simulink model "Damaper"  (R2024b)
settings: Solver=VariableStepAuto  StartTime=0.0  StopTime=10.0  RelTol=1e-3
values from neighbouring files (symbols this model uses):
  b = 10    [Damper.m]
  k = 400    [Damper.m]
  m = massValues(i)    [Damper.m]
  x0 = 1    [Damper.m]
settings Model: Creator=Ahmad  LastModifiedBy=Ahmad

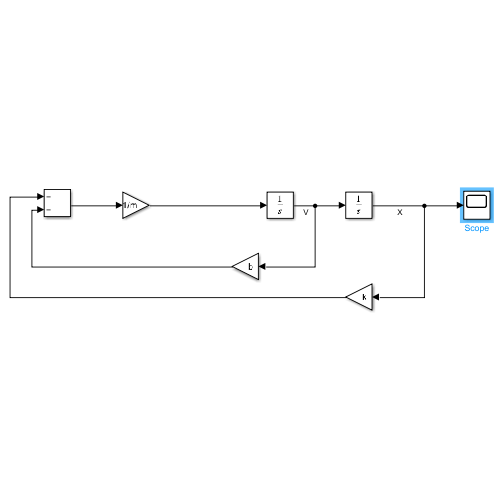
[thumbnail: Simulink's stored preview of the top-level diagram]
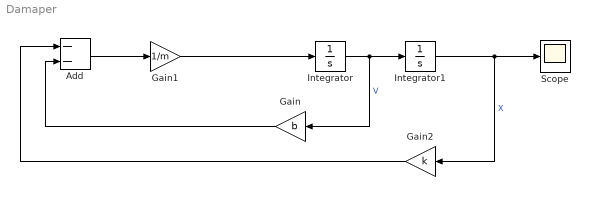
== system Damaper ==
  Add : Sum  Inputs=--
  Gain : Gain  Gain=b
  Gain1 : Gain  Gain=1/m
  Gain2 : Gain  Gain=k
  Integrator : Integrator
  Integrator1 : Integrator  InitialCondition=x0
  Scope : Scope
  wires:
  Add/1 -> Gain1/1
  Gain2/1 -> Add/1
  Gain/1 -> Add/2
  Integrator/1 -> Integrator1/1, Gain/1  "V"
  Gain1/1 -> Integrator/1
  Integrator1/1 -> Scope/1, Gain2/1  "X"
